simulink model "CubeX_LQR_3D"  (R2017b)
settings: Solver=FixedStepDiscrete  StartTime=0.0  StopTime=inf  FixedStep=Ts.base  RelTol=1e-3
PreLoadFcn:
  | waijung.modelPreload; % Required for working with Waijung Blockset. Do not remove.
InitFcn:
  | cubeparameters
  | LQR_3d
undefined symbols (not defined in the file or in its folder): deg_, g, HSEOSC, imu, K_lqr_3D, Link, LQFP176, motor, ST, STM32F417IG, Ts
libraries: simulink x29, stm32f4_i2c_lib x8, stm32f4_io_lib x7, stm32f4_adc_lib x3, stm32f4_device_config_lib x1, BC_USB x1
(part 3 of 3)

== matlab function CubeX_LQR_3D/CoG finder/MATLAB Function ==
  data: ref output; cog input
function ref = fcn(cog)

% Map over three dimensional vector to referance euler angles

rcb_tilde = cog;

rx = rcb_tilde(1); 
ry = rcb_tilde(2); 
rz = rcb_tilde(3);

psi_ref = atan2(rx, ry); 
theta_ref = atan2( sin(psi_ref)*(rx^2+ry^2),rx*rz);

ref = [ 0 ; theta_ref + deg2rad(1.5) ; psi_ref]; % Initial guess of the cog finder

== matlab function CubeX_LQR_3D/Read IMU/Accelometer Gyroscope I2C1/Read Accelometer and Gyroscope Data/Old gyro get data Used during SPI before/Take away Sensor fail reading ==
  data: y output; new input; old input
function y = fcn(new, old)
%#codegen
if(new > -257 && new < -200)
   y = old;
else
    y = new;
end

== matlab function CubeX_LQR_3D/Read IMU/Accelometer Gyroscope I2C1/Read Accelometer and Gyroscope Data/Old gyro get data Used during SPI before/Take away Sensor fail reading if two bad in raw ==
  data: y output; new input; old input
function y = fcn(new, old)
%#codegen
if(new > -257 && new < -200)
   y = old;
else
    y = new;
end

== matlab function CubeX_LQR_3D/Read IMU/Accelometer Gyroscope I2C1/Read Accelometer and Gyroscope Data/Old gyro get data Used during SPI before/Take away Sensor fail reading if two bad in raw1 ==
  data: y output; new input; old input
function y = fcn(new, old)
%#codegen
if(new > -257 && new < -200)
   y = old;
else
    y = new;
end

== matlab function CubeX_LQR_3D/Read IMU/Accelometer Gyroscope I2C1/Read Accelometer and Gyroscope Data/Old gyro get data Used during SPI before/Take away Sensor fail reading1 ==
  data: y output; new input; old input
function y = fcn(new, old)
%#codegen
if(new > -257 && new < -200)
   y = old;
else
    y = new;
end

== matlab function CubeX_LQR_3D/Read IMU/Accelometer Gyroscope I2C1/Read Accelometer and Gyroscope Data/Old gyro get data Used during SPI before/Take away Sensor fail reading if two bad in raw2 ==
  data: y output; new input; old input
function y = fcn(new, old)
%#codegen
if(new > -257 && new < -200)
   y = old;
else
    y = new;
end

== matlab function CubeX_LQR_3D/Read IMU/Accelometer Gyroscope I2C1/Read Accelometer and Gyroscope Data/Old gyro get data Used during SPI before/Take away Sensor fail reading2 ==
  data: y output; new input; old input
function y = fcn(new, old)
%#codegen
if(new > -257 && new < -200)
   y = old;
else
    y = new;
end
